simulink model "PID_scheme"  (R2018b)
settings: Solver=VariableStepAuto  StartTime=0.0  StopTime=10.0  RelTol=1e-3
model workspace (MAT data in the model file):
  N = 10
undefined symbols (not defined in the file): Kd, Ki, Kp
settings Model: Creator=alex  LastModifiedBy=alex

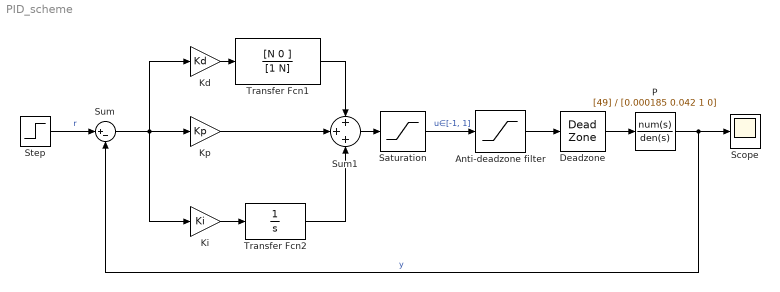
== system PID_scheme ==
  Anti-deadzone filter : Saturate
      mask Display: image('/Users/alex/Desktop/anti filter.jpeg');
  Deadzone : DeadZone  LowerValue=-50  UpperValue=50  SaturateOnIntegerOverflow=on
  "Kd " : Gain  Gain=Kd
  Ki : Gain  Gain=Ki
  Kp : Gain  Gain=Kp
  P : TransferFcn  Numerator=[49]  Denominator=[0.000185 0.042 1 0]  ContinuousStateAttributes='P'
      mask Display: image('/Users/alex/Desktop/P.png');
  Saturation : Saturate  UpperLimit=1  LowerLimit=-1
  Scope : Scope
  Step : Step  After=1000  SampleTime=0
  Sum : Sum  Inputs=|+-
  Sum1 : Sum  Inputs=+++
  Transfer Fcn1 : TransferFcn  Numerator=[N 0 ]  Denominator=[1 N]
  Transfer Fcn2 : TransferFcn  Denominator=[1 0]
  wires:
  Saturation/1 -> Anti-deadzone filter/1  "u∈[-1, 1]"
  Sum1/1 -> Saturation/1
  Step/1 -> Sum/1  "r"
  Ki/1 -> Transfer Fcn2/1
  P/1 -> Scope/1, Sum/2  "y"
  Sum/1 -> Ki/1, "Kd "/1, Kp/1
  Transfer Fcn1/1 -> Sum1/1
  Kp/1 -> Sum1/2
  Transfer Fcn2/1 -> Sum1/3
  "Kd "/1 -> Transfer Fcn1/1
  Deadzone/1 -> P/1
  Anti-deadzone filter/1 -> Deadzone/1
